simulink model "pos_test"  (R2015a)
settings: Solver=ode3  StartTime=0.0  StopTime=inf  RelTol=1e-3
libraries: arduinolib x3
settings Model: SimulationMode=external  ExtModeTrigDuration=2  Creator=shohei  LastModifiedBy=shohei
settings OptimizationCC: OptimizeModelRefInitCode=on  LifeSpan=1
settings DebuggingCC: UnderspecifiedInitializationDetection=Classic  MergeDetectMultiDrivingBlocksExec=none
settings HardwareCC: ProdBitPerInt=16  ProdBitPerPointer=8  ProdIntDivRoundTo=Zero  ProdEndianess=LittleEndian  ProdWordSize=8  ProdHWDeviceType=Atmel->AVR
settings RTWCC: SystemTargetFile=realtime.tlc  GenerateMakefile=off  TemplateMakefile=realtime.tmf  Description=Run on Target Hardware  RTWVerbose=off
settings ERTTargetCC: CombineOutputUpdateFcns=off  ExtModeTransport=3  ExtModeMexFile=ext_serial_win32_comm_rtt  ExtModeMexArgs=0 1 9600  ERTSrcFileBannerTemplate=realtime_code_template.cgt  ERTHdrFileBannerTemplate=realtime_code_template.cgt  ERTDataSrcFileTemplate=realtime_code_template.cgt  ERTDataHdrFileTemplate=realtime_code_template.cgt  ERTCustomFileTemplate=realtime_file_process.tlc

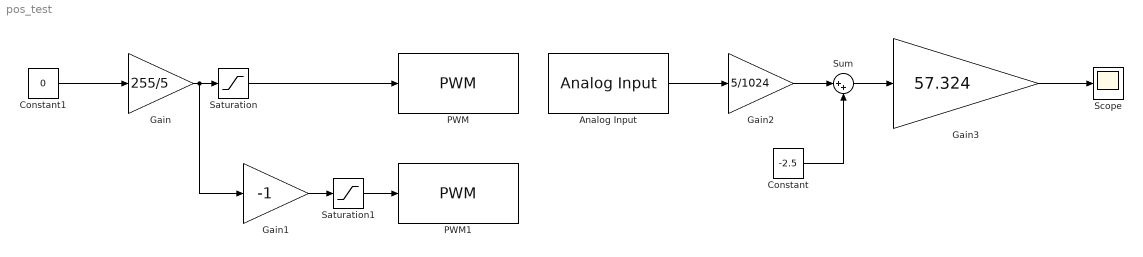
== system pos_test ==
  Analog Input : arduinolib/Analog Input  pinNumber=1  sampleTime=1  blockPlatform=arduino
  Constant : Constant  Value=-2.5
  Constant1 : Constant  Value=0
  Gain : Gain  Gain=255/5
  Gain1 : Gain  Gain=-1
  Gain2 : Gain  Gain=5/1024
  Gain3 : Gain  Gain=57.324
  PWM : arduinolib/PWM  pinNumber=3  blockPlatform=arduino
  PWM1 : arduinolib/PWM  pinNumber=5  blockPlatform=arduino
  Saturation : Saturate  UpperLimit=255  LowerLimit=0
  Saturation1 : Saturate  UpperLimit=255  LowerLimit=0
  Scope : Scope
      settings: YMin=-1.67941  YMax=-1.67941
  Sum : Sum  Inputs=|++
  wires:
  Gain/1 -> Gain1/1, Saturation/1
  Saturation/1 -> PWM/1
  Gain1/1 -> Saturation1/1
  Saturation1/1 -> PWM1/1
  Analog Input/1 -> Gain2/1
  Gain2/1 -> Sum/1
  Constant/1 -> Sum/2
  Sum/1 -> Gain3/1
  Gain3/1 -> Scope/1
  Constant1/1 -> Gain/1
